simulink model "windturbine"  (R2020a)
settings: Solver=ode4  StartTime=0.0  StopTime=10  FixedStep=10e-6  RelTol=1e-3
libraries: powerlib x16, powerlib_meascontrol x5, re_lib x1, simulink x1
settings Model: Creator=sameeraa  LastModifiedBy=vardh

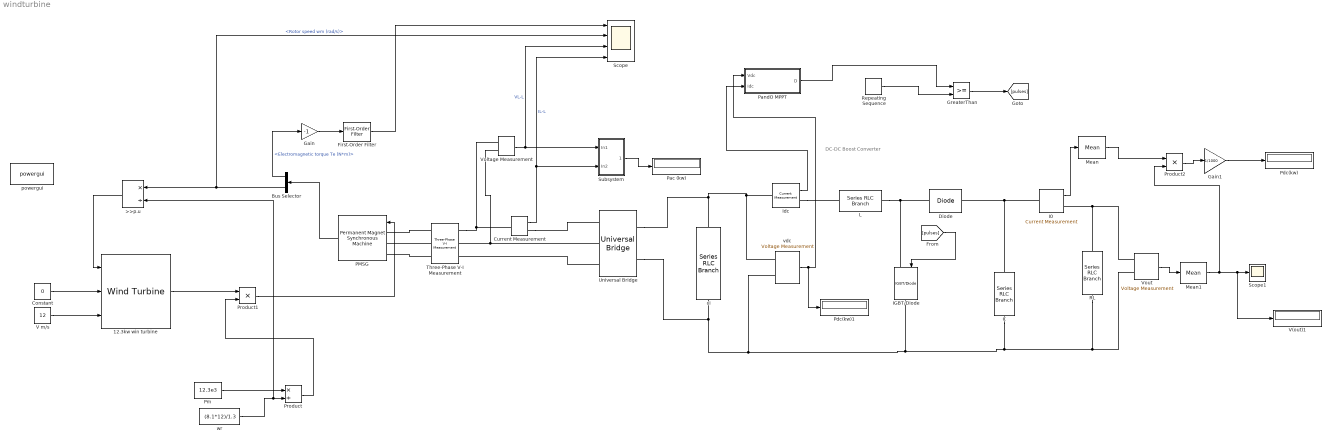
== system windturbine ==
  note: DC-DC Boost Converter
  12.3kw win turbine : re_lib/Wind Generation/Wind Turbine  Pnom=12.3e3  Pelec_base=12.3e3/0.9  wind_base=12  P_wind_base=0.85  speed_nom=1.2  pitch_angle=0  c1_c6="[0.51763          116          0.4            5           21     0.006795]"  cp_nom=0.48  lambda_nom=8.1
      settings: SourceProductBaseCode=PS
  >>p.u : Product  Inputs=*/
  Bus Selector : BusSelector  OutputSignals=Electromagnetic torque Te (N*m),Rotor speed wm (rad/s)
  C : powerlib/Elements/Series RLC Branch  LConnTagsString=__new0  RConnTagsString=__new0  BranchType=RC  Resistance=0.005  Inductance=1e-3  SetiL0=off  InitialCurrent=0  Capacitance=6.6094e-4  Setx0=off  InitialVoltage=0  Measurements=None
  Constant : Constant  Value=0
  Current Measurement : powerlib/Measurements/Current Measurement  PhasorSimulation=off  OutputType=Complex  PSBequivalent=0
  Diode : powerlib/Power Electronics/Diode  Ron=0.001  Lon=0  Vf=0.8  IC=0  UseSnubber=0  Rs=inf  Cs=inf  Measurements=off
  First-Order Filter : powerlib_meascontrol/Filters/First-Order Filter  FilterType=Lowpass  Tc=10e-3  Ts=50e-6  Initialize=on  Vac_Init=[0, 0, 50]  Vdc_Init=0  PlotResponse=off  FreqRange="[0,  200,  1]"
  Gain : Gain  Gain=-1
  Gain1 : Gain  Gain=1/1000
  GreaterThan : RelationalOperator  OutDataTypeStr=boolean  RndMeth=Simplest
  I0 : powerlib/Measurements/Current Measurement  PhasorSimulation=off  OutputType=Complex  PSBequivalent=0
  IGBT/Diode : powerlib/Power Electronics/IGBT//Diode  Ron=1e-3  Rs=1e5  Cs=inf  Measurements=off
  Idc : powerlib/Measurements/Current Measurement  PhasorSimulation=off  OutputType=Complex  PSBequivalent=0
  L : powerlib/Elements/Series RLC Branch  LConnTagsString=__new0  RConnTagsString=__new0  BranchType=L  Resistance=1  Inductance=4.5573e-05  SetiL0=off  InitialCurrent=0  Capacitance=1e-6  Setx0=off  InitialVoltage=0  Measurements=None
  Mean : powerlib_meascontrol/Measurements/Mean  Freq=60  Vinit=0  Ts=50e-6
  Mean1 : powerlib_meascontrol/Measurements/Mean  Freq=60  Vinit=0  Ts=50e-6
  PMSG : powerlib/Machines/Permanent Magnet Synchronous Machine  NbPhases=3  FluxDistribution=Sinusoidal  RotorType=Salient-pole  MechanicalLoad=Torque Tm  PresetModel=No  ShowDetailedParameters=on  MeasurementBus=off  Resistance=0.0485  Inductance=8.5e-3  dqInductances=[0.395e-3,0.395e-3]  La=0.000395  MachineConstant=Flux linkage established by magnets (V.s)  Flux=0.1194  VoltageCst=86.6271  TorqueCst=0.7164  Flat=120  Mechanical=[0.0027 0.0004924 4 0]  PolePairs=4  InitialConditions=[0,0, 0,0]  InitialConditions5ph=[0 0 0 0 0 0]  RefAngle=90 degrees behind phase A axis (modified Park)  IterativeDiscreteModel=Trapezoidal non iterative  TsBlock=-1  TsPowergui=0
  Pac (kw) : Display
  PandO MPPT : Subsystem
  Pdc(kw) : Display
  Pdc(kw)1 : Display
  Pm : Constant  Value=12.3e3
  Product : Product  Inputs=*/
  Product1 : Product
  Product2 : Product
  RL : powerlib/Elements/Series RLC Branch  LConnTagsString=__new0  RConnTagsString=__new0  BranchType=R  Resistance=13.5  Inductance=4.5  SetiL0=off  InitialCurrent=0  Capacitance=1e-6  Setx0=off  InitialVoltage=0  Measurements=None
  Repeating Sequence : simulink/Sources/Repeating Sequence  rep_seq_t=[0 1/20000]  rep_seq_y=[0 0.9]
  Scope : Scope  NumInputPorts=4
  Scope1 : Scope
  Subsystem : Subsystem
  Three-Phase V-I Measurement : powerlib/Measurements/Three-Phase V-I Measurement  VoltageMeasurement=no  SetLabelV=off  LabelV=Vabc  Vpu=off  VpuLL=off  CurrentMeasurement=no  SetLabelI=off  LabelI=Iabc  Ipu=off  Pbase=100e6  Vbase=500e3  OutputType=Complex  PhasorSimulation=off  PSBequivalent=0
  Universal Bridge : powerlib/Power Electronics/Universal Bridge  Arms=3  SnubberResistance=1e5  SnubberCapacitance=inf  Device=Diodes  Ron=1e-3  Lon=0  ForwardVoltages="[  0  0  ]"  ForwardVoltage=0  GTOparameters=[ 10e-6 , 20e-6 ]  IGBTparameters=[ 1e-6 , 2e-6 ]  Measurements=None  Measurements_2=None  converterType=Rectifier
  V m/s : Constant  Value=12
  V(out)1 : Display
      settings: Format=bank
  Voltage Measurement : powerlib/Measurements/Voltage Measurement  PhasorSimulation=off  OutputType=Complex  PSBequivalent=0
  Vout : powerlib/Measurements/Voltage Measurement  PhasorSimulation=off  OutputType=Complex  PSBequivalent=0
  ci : powerlib/Elements/Series RLC Branch  LConnTagsString=__new0  RConnTagsString=__new0  BranchType=RC  Resistance=0.005  Inductance=1e-3  SetiL0=off  InitialCurrent=0  Capacitance=6.6094e-4  Setx0=off  InitialVoltage=0  Measurements=None
  powergui : powerlib/powergui  Priority=1  SimulationMode=Continuous  SampleTime=20e-6  frequency=60  Iterations=50  frequencyindice=0  Pbase=100e6  ErrMax=1e-4  UnitsV=kV  UnitsW=MW  buscounter=0  FunctionMessages=off  echomessages=off  EnableUseOfTLC=off  CurrentSourceSwitches=off  DisableSnubberDevices=off  DisableRonSwitches=off  DisableVfSwitches=off  DisplayEquations=off  AutomaticDiscreteSolvers=off  SolverType=Tustin/Backward Euler (TBE)  Interpol=off  ExternalGateDelay=off  methode=off  Ts=100  x0status=blocks  SPID=on  SwTol=0  HookPort=off  NonlinearTolerance=1e-4  nMaxIteration=100  ContinueOnMaxIteration=off  RestoreLinks=warning  ResistiveCurrentMeasurement=off  Frange=[0:2:500]  Ylog=off  Xlog=on  ShowGrid=off  save=off  variable=ZData  structure=0  ZoomFFT=off  StartTime=0.0  cycles=1  DisplayStyle=1  fundamental=60  FreqAxis=off  MaxFrequency=1000  frequencyindicesteady=1  RmsSteady=1  display=off
  vdc : powerlib/Measurements/Voltage Measurement  PhasorSimulation=off  OutputType=Complex  PSBequivalent=0
  wr : Constant  Value=(8.1*12)/1.3
  wires:
  Constant/1 -> 12.3kw win turbine/2
  V m/s/1 -> 12.3kw win turbine/3
  12.3kw win turbine/1 -> Product1/1
  Pm/1 -> Product/1
  wr/1 -> >>p.u/2, Product/2
  Product/1 -> Product1/2
  Product1/1 -> PMSG/1
  PMSG/1 -> Bus Selector/1
  Bus Selector/2 -> >>p.u/1, Scope/2  "<Rotor speed wm (rad/s)>"
  >>p.u/1 -> 12.3kw win turbine/1
  First-Order Filter/1 -> Scope/1
  Bus Selector/1 -> Gain/1  "<Electromagnetic torque Te (N*m)>"
  Gain/1 -> First-Order Filter/1
  Voltage Measurement/1 -> Scope/3, Subsystem/1(In1)  "VL-L"
  Current Measurement/1 -> Scope/4, Subsystem/2(In2)  "IL-L"
  Subsystem/1(Out1) -> Pac (kw)/1
  vdc/1 -> PandO MPPT/1(Vdc), Pdc(kw)1/1
  Idc/1 -> PandO MPPT/2(Idc)
  Repeating Sequence/1 -> GreaterThan/2
  PandO MPPT/1(D) -> GreaterThan/1
  GreaterThan/1 -> [pulses]
  I0/1 -> Mean/1
  Vout/1 -> Mean1/1
  Mean/1 -> Product2/1
  Mean1/1 -> Product2/2, V(out)1/1, Scope1/1
  Product2/1 -> Gain1/1
  Gain1/1 -> Pdc(kw)/1
  [pulses] -> IGBT/Diode/1
  connections:
  Three-Phase V-I Measurement/LConn1 -- PMSG/LConn1
  Three-Phase V-I Measurement/LConn2 -- PMSG/LConn2
  Three-Phase V-I Measurement/LConn3 -- PMSG/LConn3
  Three-Phase V-I Measurement/RConn1 -- Voltage Measurement/LConn1 -- Current Measurement/LConn1
  Universal Bridge/LConn2 -- Voltage Measurement/LConn2 -- Three-Phase V-I Measurement/RConn2
  Universal Bridge/LConn3 -- Three-Phase V-I Measurement/RConn3
  Current Measurement/RConn1 -- Universal Bridge/LConn1
  Universal Bridge/RConn2 -- vdc/LConn2 -- Vout/LConn2 -- RL/RConn1 -- C/RConn1 -- IGBT/Diode/RConn1 -- ci/RConn1
  Universal Bridge/RConn1 -- vdc/LConn1 -- Idc/LConn1 -- ci/LConn1
  Idc/RConn1 -- L/LConn1
  L/RConn1 -- Diode/LConn1 -- IGBT/Diode/LConn1
  RL/LConn1 -- Vout/LConn1 -- I0/RConn1
  I0/LConn1 -- C/LConn1 -- Diode/RConn1

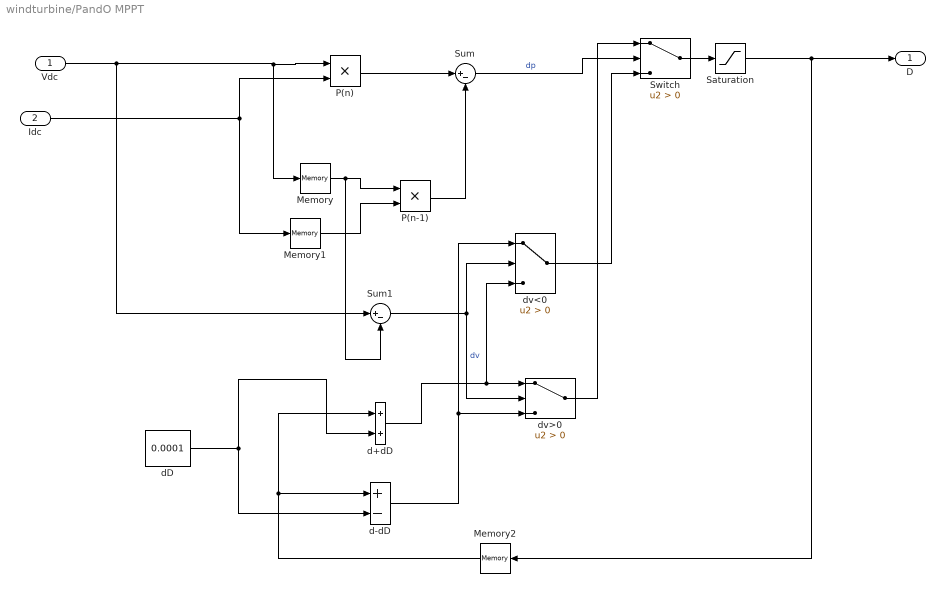
== system windturbine/PandO MPPT ==
  Vdc : Inport
  Idc : Inport  Port=2
  Memory : Memory  InheritSampleTime=on
  Memory1 : Memory  InheritSampleTime=on
  Memory2 : Memory  InheritSampleTime=on
  P(n) : Product
  P(n-1) : Product
  Saturation : Saturate  UpperLimit=inf
  Sum : Sum  Inputs=|+-
  Sum1 : Sum  Inputs=|+-
  Switch : Switch  Criteria=u2 > Threshold
  d+dD : Sum
  d-dD : Sum  Inputs=+-
  dD : Constant  Value=0.0001
  dv<0 : Switch  Criteria=u2 > Threshold
  dv>0 : Switch  Criteria=u2 > Threshold
  D : Outport
  wires:
  Idc/1 -> P(n)/2, Memory1/1
  Memory/1 -> Sum1/2, P(n-1)/1
  Memory1/1 -> P(n-1)/2
  P(n)/1 -> Sum/1
  P(n-1)/1 -> Sum/2
  Vdc/1 -> Sum1/1, Memory/1, P(n)/1
  Sum1/1 -> dv>0/2, dv<0/2  "dv"
  Sum/1 -> Switch/2  "dp"
  Switch/1 -> Saturation/1
  Memory2/1 -> d+dD/1, d-dD/1
  dD/1 -> d+dD/2, d-dD/2
  d-dD/1 -> dv>0/3, dv<0/1
  d+dD/1 -> dv<0/3, dv>0/1
  dv<0/1 -> Switch/3
  dv>0/1 -> Switch/1
  Saturation/1 -> Memory2/1, D/1

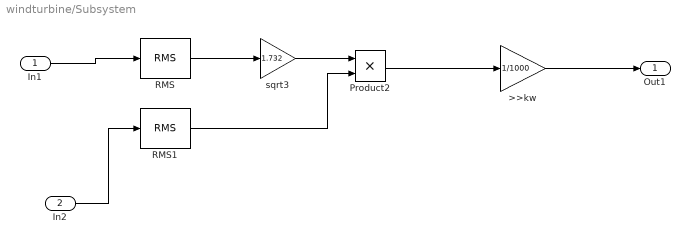
== system windturbine/Subsystem ==
  In1 : Inport
  In2 : Inport  Port=2
  >>kw : Gain  Gain=1/1000
  Product2 : Product
  RMS : powerlib_meascontrol/Measurements/RMS  TrueRMS=on  Freq=50  RMSInit=120  Ts=50e-6
  RMS1 : powerlib_meascontrol/Measurements/RMS  TrueRMS=on  Freq=60  RMSInit=120  Ts=0
      link override TrueRMS /Mean value/Model/integrator: InitialCondition=1
  sqrt3 : Gain  Gain=1.732
  Out1 : Outport
  wires:
  sqrt3/1 -> Product2/1
  RMS/1 -> sqrt3/1
  RMS1/1 -> Product2/2
  In2/1 -> RMS1/1
  In1/1 -> RMS/1
  >>kw/1 -> Out1/1
  Product2/1 -> >>kw/1
